simulink model "SimulacionTanqueControlado"  (R2020a)
settings: Solver=VariableStepAuto  StartTime=0.0  StopTime=tsim  RelTol=1e-3
values from neighbouring files (symbols this model uses):
  Qi = 4    [LQRTanque.m]
  Ti = 49.9    [LQRTanque.m]
  tmuestra = 0.5    [GeneracionDatosTanque.m]    (also in LQRTanque.m; SimulacionTanque.m)
  Ui = resul(11:12)    [LQRTanque.m]
  Yr = [5; 67]    [LQRTanque.m]
undefined symbols (not defined in the file or in its folder): alpha, Area, ControlDiscretoRealimentado, K1, K2, Kp, T1, T2, tau1, tau2, tdelay1, tdelay2, tdelayQ, Te
settings Model: Creator=pablo  LastModifiedBy=pablo
settings DataIOCC: SaveOutput=off  SignalLogging=off  DSMLogging=off  SaveTime=off  ReturnWorkspaceOutputs=off
settings DebuggingCC: UnderSpecifiedDimensionMsg=warning  ArithmeticOperatorsInVariantConditions=warning
settings SFSimCC: CustomCodeUndefinedFunction=UseInterfaceOnly

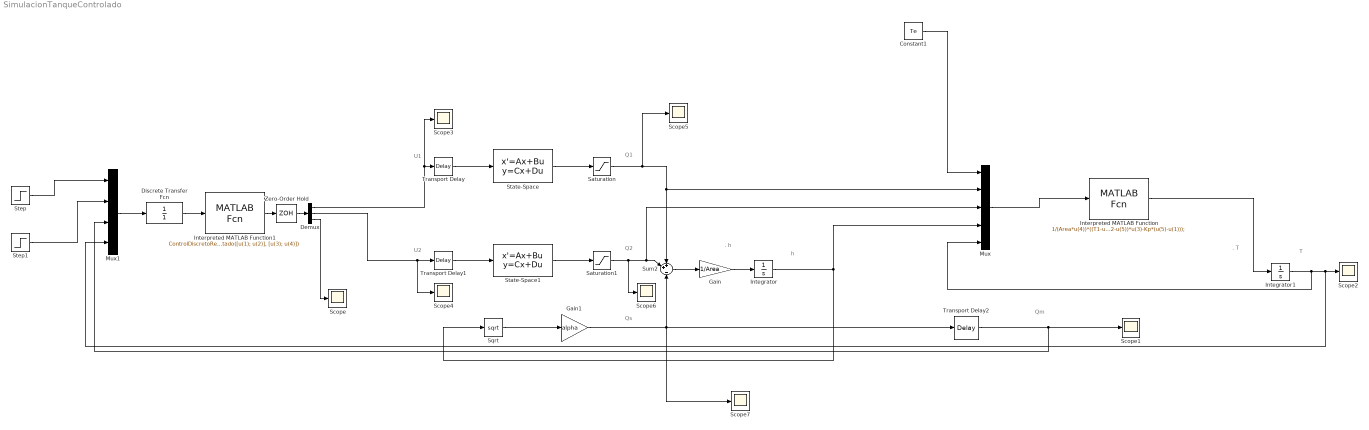
== system SimulacionTanqueControlado ==
  note: Qm
  note: .
      | T
  note: T
  note: h
  note: .
      |  h
  note: Qs
  note: Q1
  note: U1
  note: Q2
  note: U2
  Constant1 : Constant  Value=Te
  Demux : Demux  Outputs=[1 1 2]
  Discrete Transfer Fcn : DiscreteTransferFcn  Numerator=1  Denominator=1  SampleTime=tmuestra
  Gain : Gain  Gain=1/Area
  Gain1 : Gain  Gain=alpha
  Integrator : Integrator  InitialCondition=(Qi/alpha^2)  LimitOutput=on  LowerSaturationLimit=0
  Integrator1 : Integrator  InitialCondition=Ti  LowerSaturationLimit=0
  Interpreted MATLAB Function : MATLABFcn  MATLABFcn=1/(Area*u(4))*((T1-u(5))*u(2)+(T2-u(5))*u(3)-Kp*(u(5)-u(1)));  OutputDimensions=1
  Interpreted MATLAB Function1 : MATLABFcn  MATLABFcn=ControlDiscretoRealimentado([u(1); u(2)], [u(3); u(4)])  OutputDimensions=4
  Mux : Mux  Inputs=5
  Mux1 : Mux
  Saturation : Saturate  UpperLimit=inf  LowerLimit=0
  Saturation1 : Saturate  UpperLimit=inf  LowerLimit=0
  Scope{,1..7} (8 alike) : Scope
  Sqrt : Sqrt  SaturateOnIntegerOverflow=on
  State-Space : StateSpace  A=-1/tau1  B=K1/tau1  D=0  InitialCondition=2
  State-Space1 : StateSpace  A=-1/tau2  B=K2/tau2  D=0  InitialCondition=2
  Step : Step  Time=10  Before=Qi  After=Yr(1)  SampleTime=tmuestra
  Step1 : Step  Time=10  Before=Ti  After=Yr(2)  SampleTime=tmuestra
  Sum2 : Sum  Inputs=++|-
  Transport Delay : TransportDelay  DelayTime=tdelay1  InitialOutput=Ui(1)
  Transport Delay1 : TransportDelay  DelayTime=tdelay2  InitialOutput=Ui(2)
  Transport Delay2 : TransportDelay  DelayTime=tdelayQ  InitialOutput=Qi
  Zero-Order Hold : ZeroOrderHold  SampleTime=tmuestra
  wires:
  Demux/1 -> Scope3/1, Transport Delay/1
  Transport Delay/1 -> State-Space/1
  State-Space/1 -> Saturation/1
  Transport Delay1/1 -> State-Space1/1
  State-Space1/1 -> Saturation1/1
  Demux/2 -> Scope4/1, Transport Delay1/1
  Sum2/1 -> Gain/1
  Gain1/1 -> Scope7/1, Sum2/3, Transport Delay2/1
  Sqrt/1 -> Gain1/1
  Gain/1 -> Integrator/1
  Integrator/1 -> Sqrt/1, Mux/4
  Saturation/1 -> Scope5/1, Mux/2, Sum2/1
  Saturation1/1 -> Scope6/1, Mux/3, Sum2/2
  Constant1/1 -> Mux/1
  Integrator1/1 -> Mux/5, Mux1/4, Scope2/1
  Transport Delay2/1 -> Mux1/3, Scope1/1
  Step/1 -> Mux1/1
  Step1/1 -> Mux1/2
  Demux/3 -> Scope/1
  Mux1/1 -> Discrete Transfer Fcn/1
  Discrete Transfer Fcn/1 -> Interpreted MATLAB Function1/1
  Interpreted MATLAB Function1/1 -> Zero-Order Hold/1
  Zero-Order Hold/1 -> Demux/1
  Interpreted MATLAB Function/1 -> Integrator1/1
  Mux/1 -> Interpreted MATLAB Function/1
